simulink model "snap_fengine"  (R2016b)
settings: Solver=VariableStepDiscrete  StartTime=0.0  StopTime=10.0  RelTol=1e-3
libraries: xbsIndex_r4 x4489, casper_library_misc x36, xps_library x10, casper_library_sources x6, casper_library_delays x5, casper_library_reorder x2, casper_library_communications x1
(part 13 of 38)

== system snap_fengine/rotator/rotator3 ==
  din : Inport
  phase : Inport  Port=2
  "CORDIC 6.0 " : xbsIndex_r4/CORDIC 6.0   functional_selection=Rotate  architectural_configuration=Parallel  pipelining_mode=Optimal  data_format=SignedFraction  phase_format=Radians  input_width=18  output_width=18  round_mode=Nearest_Even  iterations=0  precision=0  compensation_scaling=No_Scale_Compensation  coarse_rotation=off  aclken=off  aresetn=off  out_tready=off  cartesian_has_tuser=off  cartesian_has_tlast=off  cartesian_tuser_width=1  phase_has_tuser=off  phase_has_tlast=off  phase_tuser_width=1  out_tlast_behv=Null  flow_control=NonBlocking  optimize_goal=Resources  trim_axipin_name=on  simulation_type=hybrid_sim  simulation_model=sysgen:cordic_v6_0  data_path_portlist={'s_axis_cartesian_tdata_imag', 's_axis_cartesian_tdata_real', 's_axis_phase_tdata_phase', 'm_axis_dout_tdata_imag', 'm_axis_dout_tdata_real', 'm_axis_dout_tdata_phase','m_axis_dout_tdata'}  ip_name=CORDIC  ip_version=6.0  dsptool_ready=true  ipcore_usecache=true  ipcore_useipmodelcache=true  wrapper_available=true  port_translation_map={ 'aclken' => 'en', 'aresetn' => 'rst' }  block_type=cordic_v6_0
      settings: infoedit=CORDIC 6.0
  Constant2 : xbsIndex_r4/Constant  const=1  gui_display_data_type=Boolean  arith_type=Boolean  n_bits=32  bin_pt=0  preci_type=Single  exp_width=8  frac_width=24  explicit_period=on  period=1  equ=P=C  opselect=C  inp2=PCIN>>17  opr=+  inp1=P  carry=CIN  dbl_ovrd=off  block_type=constant
  Constant3 : xbsIndex_r4/Constant  const=1  gui_display_data_type=Boolean  arith_type=Boolean  n_bits=32  bin_pt=0  preci_type=Single  exp_width=8  frac_width=24  explicit_period=on  period=1  equ=P=C  opselect=C  inp2=PCIN>>17  opr=+  inp1=P  carry=CIN  dbl_ovrd=off  block_type=constant
  Reinterpret : xbsIndex_r4/Reinterpret  force_arith_type=on  arith_type="Signed  (2's comp)"  force_bin_pt=on  bin_pt=16  block_type=reinterpret
  Reinterpret1 : xbsIndex_r4/Reinterpret  force_arith_type=on  arith_type="Signed  (2's comp)"  force_bin_pt=on  bin_pt=16  block_type=reinterpret
  c_to_ri : casper_library_misc/c_to_ri  n_bits=18  bin_pt=17
  ri_to_c : casper_library_misc/ri_to_c
  vld : Outport
  dout : Outport  Port=2
  wires:
  Constant2/1 -> "CORDIC 6.0 "/4
  c_to_ri/1 -> Reinterpret/1
  ri_to_c/1 -> dout/1
  phase/1 -> "CORDIC 6.0 "/5
  Constant3/1 -> "CORDIC 6.0 "/1
  "CORDIC 6.0 "/2 -> ri_to_c/2
  "CORDIC 6.0 "/1 -> vld/1
  "CORDIC 6.0 "/3 -> ri_to_c/1
  din/1 -> c_to_ri/1
  c_to_ri/2 -> Reinterpret1/1
  Reinterpret/1 -> "CORDIC 6.0 "/3
  Reinterpret1/1 -> "CORDIC 6.0 "/2

== system snap_fengine/rotator/rotator4 ==
  din : Inport
  phase : Inport  Port=2
  "CORDIC 6.0 " : xbsIndex_r4/CORDIC 6.0   functional_selection=Rotate  architectural_configuration=Parallel  pipelining_mode=Optimal  data_format=SignedFraction  phase_format=Radians  input_width=18  output_width=18  round_mode=Nearest_Even  iterations=0  precision=0  compensation_scaling=No_Scale_Compensation  coarse_rotation=off  aclken=off  aresetn=off  out_tready=off  cartesian_has_tuser=off  cartesian_has_tlast=off  cartesian_tuser_width=1  phase_has_tuser=off  phase_has_tlast=off  phase_tuser_width=1  out_tlast_behv=Null  flow_control=NonBlocking  optimize_goal=Resources  trim_axipin_name=on  simulation_type=hybrid_sim  simulation_model=sysgen:cordic_v6_0  data_path_portlist={'s_axis_cartesian_tdata_imag', 's_axis_cartesian_tdata_real', 's_axis_phase_tdata_phase', 'm_axis_dout_tdata_imag', 'm_axis_dout_tdata_real', 'm_axis_dout_tdata_phase','m_axis_dout_tdata'}  ip_name=CORDIC  ip_version=6.0  dsptool_ready=true  ipcore_usecache=true  ipcore_useipmodelcache=true  wrapper_available=true  port_translation_map={ 'aclken' => 'en', 'aresetn' => 'rst' }  block_type=cordic_v6_0
      settings: infoedit=CORDIC 6.0
  Constant2 : xbsIndex_r4/Constant  const=1  gui_display_data_type=Boolean  arith_type=Boolean  n_bits=32  bin_pt=0  preci_type=Single  exp_width=8  frac_width=24  explicit_period=on  period=1  equ=P=C  opselect=C  inp2=PCIN>>17  opr=+  inp1=P  carry=CIN  dbl_ovrd=off  block_type=constant
  Constant3 : xbsIndex_r4/Constant  const=1  gui_display_data_type=Boolean  arith_type=Boolean  n_bits=32  bin_pt=0  preci_type=Single  exp_width=8  frac_width=24  explicit_period=on  period=1  equ=P=C  opselect=C  inp2=PCIN>>17  opr=+  inp1=P  carry=CIN  dbl_ovrd=off  block_type=constant
  Reinterpret : xbsIndex_r4/Reinterpret  force_arith_type=on  arith_type="Signed  (2's comp)"  force_bin_pt=on  bin_pt=16  block_type=reinterpret
  Reinterpret1 : xbsIndex_r4/Reinterpret  force_arith_type=on  arith_type="Signed  (2's comp)"  force_bin_pt=on  bin_pt=16  block_type=reinterpret
  c_to_ri : casper_library_misc/c_to_ri  n_bits=18  bin_pt=17
  ri_to_c : casper_library_misc/ri_to_c
  vld : Outport
  dout : Outport  Port=2
  wires:
  Reinterpret1/1 -> "CORDIC 6.0 "/2
  Reinterpret/1 -> "CORDIC 6.0 "/3
  c_to_ri/2 -> Reinterpret1/1
  din/1 -> c_to_ri/1
  "CORDIC 6.0 "/3 -> ri_to_c/1
  "CORDIC 6.0 "/1 -> vld/1
  "CORDIC 6.0 "/2 -> ri_to_c/2
  Constant3/1 -> "CORDIC 6.0 "/1
  phase/1 -> "CORDIC 6.0 "/5
  ri_to_c/1 -> dout/1
  c_to_ri/1 -> Reinterpret/1
  Constant2/1 -> "CORDIC 6.0 "/4

== system snap_fengine/rotator/rotator5 ==
  din : Inport
  phase : Inport  Port=2
  "CORDIC 6.0 " : xbsIndex_r4/CORDIC 6.0   functional_selection=Rotate  architectural_configuration=Parallel  pipelining_mode=Optimal  data_format=SignedFraction  phase_format=Radians  input_width=18  output_width=18  round_mode=Nearest_Even  iterations=0  precision=0  compensation_scaling=No_Scale_Compensation  coarse_rotation=off  aclken=off  aresetn=off  out_tready=off  cartesian_has_tuser=off  cartesian_has_tlast=off  cartesian_tuser_width=1  phase_has_tuser=off  phase_has_tlast=off  phase_tuser_width=1  out_tlast_behv=Null  flow_control=NonBlocking  optimize_goal=Resources  trim_axipin_name=on  simulation_type=hybrid_sim  simulation_model=sysgen:cordic_v6_0  data_path_portlist={'s_axis_cartesian_tdata_imag', 's_axis_cartesian_tdata_real', 's_axis_phase_tdata_phase', 'm_axis_dout_tdata_imag', 'm_axis_dout_tdata_real', 'm_axis_dout_tdata_phase','m_axis_dout_tdata'}  ip_name=CORDIC  ip_version=6.0  dsptool_ready=true  ipcore_usecache=true  ipcore_useipmodelcache=true  wrapper_available=true  port_translation_map={ 'aclken' => 'en', 'aresetn' => 'rst' }  block_type=cordic_v6_0
      settings: infoedit=CORDIC 6.0
  Constant2 : xbsIndex_r4/Constant  const=1  gui_display_data_type=Boolean  arith_type=Boolean  n_bits=32  bin_pt=0  preci_type=Single  exp_width=8  frac_width=24  explicit_period=on  period=1  equ=P=C  opselect=C  inp2=PCIN>>17  opr=+  inp1=P  carry=CIN  dbl_ovrd=off  block_type=constant
  Constant3 : xbsIndex_r4/Constant  const=1  gui_display_data_type=Boolean  arith_type=Boolean  n_bits=32  bin_pt=0  preci_type=Single  exp_width=8  frac_width=24  explicit_period=on  period=1  equ=P=C  opselect=C  inp2=PCIN>>17  opr=+  inp1=P  carry=CIN  dbl_ovrd=off  block_type=constant
  Reinterpret : xbsIndex_r4/Reinterpret  force_arith_type=on  arith_type="Signed  (2's comp)"  force_bin_pt=on  bin_pt=16  block_type=reinterpret
  Reinterpret1 : xbsIndex_r4/Reinterpret  force_arith_type=on  arith_type="Signed  (2's comp)"  force_bin_pt=on  bin_pt=16  block_type=reinterpret
  c_to_ri : casper_library_misc/c_to_ri  n_bits=18  bin_pt=17
  ri_to_c : casper_library_misc/ri_to_c
  vld : Outport
  dout : Outport  Port=2
  wires:
  Constant2/1 -> "CORDIC 6.0 "/4
  c_to_ri/1 -> Reinterpret/1
  ri_to_c/1 -> dout/1
  phase/1 -> "CORDIC 6.0 "/5
  Constant3/1 -> "CORDIC 6.0 "/1
  "CORDIC 6.0 "/2 -> ri_to_c/2
  "CORDIC 6.0 "/1 -> vld/1
  "CORDIC 6.0 "/3 -> ri_to_c/1
  din/1 -> c_to_ri/1
  c_to_ri/2 -> Reinterpret1/1
  Reinterpret/1 -> "CORDIC 6.0 "/3
  Reinterpret1/1 -> "CORDIC 6.0 "/2

== system snap_fengine/rotator/rotator6 ==
  din : Inport
  phase : Inport  Port=2
  "CORDIC 6.0 " : xbsIndex_r4/CORDIC 6.0   functional_selection=Rotate  architectural_configuration=Parallel  pipelining_mode=Optimal  data_format=SignedFraction  phase_format=Radians  input_width=18  output_width=18  round_mode=Nearest_Even  iterations=0  precision=0  compensation_scaling=No_Scale_Compensation  coarse_rotation=off  aclken=off  aresetn=off  out_tready=off  cartesian_has_tuser=off  cartesian_has_tlast=off  cartesian_tuser_width=1  phase_has_tuser=off  phase_has_tlast=off  phase_tuser_width=1  out_tlast_behv=Null  flow_control=NonBlocking  optimize_goal=Resources  trim_axipin_name=on  simulation_type=hybrid_sim  simulation_model=sysgen:cordic_v6_0  data_path_portlist={'s_axis_cartesian_tdata_imag', 's_axis_cartesian_tdata_real', 's_axis_phase_tdata_phase', 'm_axis_dout_tdata_imag', 'm_axis_dout_tdata_real', 'm_axis_dout_tdata_phase','m_axis_dout_tdata'}  ip_name=CORDIC  ip_version=6.0  dsptool_ready=true  ipcore_usecache=true  ipcore_useipmodelcache=true  wrapper_available=true  port_translation_map={ 'aclken' => 'en', 'aresetn' => 'rst' }  block_type=cordic_v6_0
      settings: infoedit=CORDIC 6.0
  Constant2 : xbsIndex_r4/Constant  const=1  gui_display_data_type=Boolean  arith_type=Boolean  n_bits=32  bin_pt=0  preci_type=Single  exp_width=8  frac_width=24  explicit_period=on  period=1  equ=P=C  opselect=C  inp2=PCIN>>17  opr=+  inp1=P  carry=CIN  dbl_ovrd=off  block_type=constant
  Constant3 : xbsIndex_r4/Constant  const=1  gui_display_data_type=Boolean  arith_type=Boolean  n_bits=32  bin_pt=0  preci_type=Single  exp_width=8  frac_width=24  explicit_period=on  period=1  equ=P=C  opselect=C  inp2=PCIN>>17  opr=+  inp1=P  carry=CIN  dbl_ovrd=off  block_type=constant
  Reinterpret : xbsIndex_r4/Reinterpret  force_arith_type=on  arith_type="Signed  (2's comp)"  force_bin_pt=on  bin_pt=16  block_type=reinterpret
  Reinterpret1 : xbsIndex_r4/Reinterpret  force_arith_type=on  arith_type="Signed  (2's comp)"  force_bin_pt=on  bin_pt=16  block_type=reinterpret
  c_to_ri : casper_library_misc/c_to_ri  n_bits=18  bin_pt=17
  ri_to_c : casper_library_misc/ri_to_c
  vld : Outport
  dout : Outport  Port=2
  wires:
  Constant2/1 -> "CORDIC 6.0 "/4
  c_to_ri/1 -> Reinterpret/1
  ri_to_c/1 -> dout/1
  phase/1 -> "CORDIC 6.0 "/5
  Constant3/1 -> "CORDIC 6.0 "/1
  "CORDIC 6.0 "/2 -> ri_to_c/2
  "CORDIC 6.0 "/1 -> vld/1
  "CORDIC 6.0 "/3 -> ri_to_c/1
  din/1 -> c_to_ri/1
  c_to_ri/2 -> Reinterpret1/1
  Reinterpret/1 -> "CORDIC 6.0 "/3
  Reinterpret1/1 -> "CORDIC 6.0 "/2

== system snap_fengine/rotator/rotator7 ==
  din : Inport
  phase : Inport  Port=2
  "CORDIC 6.0 " : xbsIndex_r4/CORDIC 6.0   functional_selection=Rotate  architectural_configuration=Parallel  pipelining_mode=Optimal  data_format=SignedFraction  phase_format=Radians  input_width=18  output_width=18  round_mode=Nearest_Even  iterations=0  precision=0  compensation_scaling=No_Scale_Compensation  coarse_rotation=off  aclken=off  aresetn=off  out_tready=off  cartesian_has_tuser=off  cartesian_has_tlast=off  cartesian_tuser_width=1  phase_has_tuser=off  phase_has_tlast=off  phase_tuser_width=1  out_tlast_behv=Null  flow_control=NonBlocking  optimize_goal=Resources  trim_axipin_name=on  simulation_type=hybrid_sim  simulation_model=sysgen:cordic_v6_0  data_path_portlist={'s_axis_cartesian_tdata_imag', 's_axis_cartesian_tdata_real', 's_axis_phase_tdata_phase', 'm_axis_dout_tdata_imag', 'm_axis_dout_tdata_real', 'm_axis_dout_tdata_phase','m_axis_dout_tdata'}  ip_name=CORDIC  ip_version=6.0  dsptool_ready=true  ipcore_usecache=true  ipcore_useipmodelcache=true  wrapper_available=true  port_translation_map={ 'aclken' => 'en', 'aresetn' => 'rst' }  block_type=cordic_v6_0
      settings: infoedit=CORDIC 6.0
  Constant2 : xbsIndex_r4/Constant  const=1  gui_display_data_type=Boolean  arith_type=Boolean  n_bits=32  bin_pt=0  preci_type=Single  exp_width=8  frac_width=24  explicit_period=on  period=1  equ=P=C  opselect=C  inp2=PCIN>>17  opr=+  inp1=P  carry=CIN  dbl_ovrd=off  block_type=constant
  Constant3 : xbsIndex_r4/Constant  const=1  gui_display_data_type=Boolean  arith_type=Boolean  n_bits=32  bin_pt=0  preci_type=Single  exp_width=8  frac_width=24  explicit_period=on  period=1  equ=P=C  opselect=C  inp2=PCIN>>17  opr=+  inp1=P  carry=CIN  dbl_ovrd=off  block_type=constant
  Reinterpret : xbsIndex_r4/Reinterpret  force_arith_type=on  arith_type="Signed  (2's comp)"  force_bin_pt=on  bin_pt=16  block_type=reinterpret
  Reinterpret1 : xbsIndex_r4/Reinterpret  force_arith_type=on  arith_type="Signed  (2's comp)"  force_bin_pt=on  bin_pt=16  block_type=reinterpret
  c_to_ri : casper_library_misc/c_to_ri  n_bits=18  bin_pt=17
  ri_to_c : casper_library_misc/ri_to_c
  vld : Outport
  dout : Outport  Port=2
  wires:
  Reinterpret1/1 -> "CORDIC 6.0 "/2
  Reinterpret/1 -> "CORDIC 6.0 "/3
  c_to_ri/2 -> Reinterpret1/1
  din/1 -> c_to_ri/1
  "CORDIC 6.0 "/3 -> ri_to_c/1
  "CORDIC 6.0 "/1 -> vld/1
  "CORDIC 6.0 "/2 -> ri_to_c/2
  Constant3/1 -> "CORDIC 6.0 "/1
  phase/1 -> "CORDIC 6.0 "/5
  ri_to_c/1 -> dout/1
  c_to_ri/1 -> Reinterpret/1
  Constant2/1 -> "CORDIC 6.0 "/4

== system snap_fengine/sync/arm ==
  sim_1 : Inport
  io_delay : xbsIndex_r4/Delay  rst=off  infoeditControl=Selection of Reset will increase slice count due to use of real FFs and instead of SRLs  en=off  latency=0  reg_retiming=on  dbl_ovrd=off  block_type=delay
  reint1 : xbsIndex_r4/Reinterpret  force_arith_type=on  arith_type=Unsigned  force_bin_pt=on  bin_pt=0  block_type=reinterpret
  slice_reg : xbsIndex_r4/Slice  nbits=32  boolean_output=off  mode=Lower Bit Location + Width  bit1=0  base1=MSB of Input  bit0=0  base0=LSB of Input  dbl_ovrd=off  block_type=slice
  snap_fengine_sync_arm_user_data_out : xbsIndex_r4/Gateway In  gui_display_data_type=Fixed-point  arith_type=Unsigned  n_bits=32  bin_pt=0  preci_type=Single  exp_width=8  frac_width=24  rows=1  columns=1  quantization="Round  (unbiased: +/- Inf)"  overflow=Saturate  period=1  UseAsADC=off  ADCChannel='1'  interface=None  automatic_assignment=on  address_offset=hex2dec('00')  intf_name=''  intf_description=''  default_value=0  timing_constraint=None  locs_specified=off  LOCs={}  io_standard={}  inherit_from_input=off  hdl_port=on  dbl_ovrd=off  block_type=gatewayin
  in_reg : Outport
  wires:
  snap_fengine_sync_arm_user_data_out/1 -> io_delay/1
  sim_1/1 -> snap_fengine_sync_arm_user_data_out/1
  io_delay/1 -> slice_reg/1
  slice_reg/1 -> reint1/1
  reint1/1 -> in_reg/1

== system snap_fengine/sync/count ==
  out_reg : Inport
  assert_reg : xbsIndex_r4/Assert  assert_type=on  type_source=Explicitly  gui_display_data_type=Fixed-point  arith_type=Unsigned  n_bits=32  bin_pt=0  preci_type=Single  exp_width=8  frac_width=24  assert_rate=off  rate_source=Explicitly  period=1  output_port=on  block_type=assert
  cast_gw : xbsIndex_r4/Convert  gui_display_data_type=Fixed-point  arith_type=Unsigned  n_bits=32  bin_pt=0  float_type=Single  exp_bits=8  fraction_bits=24  quantization=Truncate  overflow=Wrap  en=off  latency=1  pipeline=off  dbl_ovrd=off  block_type=convert
  io_delay : xbsIndex_r4/Delay  rst=off  infoeditControl=Selection of Reset will increase slice count due to use of real FFs and instead of SRLs  en=off  latency=0  reg_retiming=on  dbl_ovrd=off  block_type=delay
  reint1 : xbsIndex_r4/Reinterpret  force_arith_type=on  arith_type=Unsigned  force_bin_pt=on  bin_pt=0  block_type=reinterpret
  snap_fengine_sync_count_user_data_in : xbsIndex_r4/Gateway Out  inherit_from_input=off  hdl_port=on  rows=1  columns=1  UseAsDAC=off  DACChannel='1'  interface=None  automatic_assignment=on  address_offset=hex2dec('00')  intf_name=''  intf_description=''  timing_constraint=None  locs_specified=off  LOCs={}  io_standard={}  block_type=gatewayout
  sim_out : Outport
  wires:
  io_delay/1 -> cast_gw/1
  cast_gw/1 -> snap_fengine_sync_count_user_data_in/1
  snap_fengine_sync_count_user_data_in/1 -> sim_out/1
  out_reg/1 -> assert_reg/1
  assert_reg/1 -> reint1/1
  reint1/1 -> io_delay/1

== system snap_fengine/sync/ed ==
  in : Inport
  Delay : xbsIndex_r4/Delay  rst=off  infoeditControl=Selection of Reset will increase slice count due to use of real FFs and instead of SRLs  en=off  latency=1  reg_retiming=off  dbl_ovrd=off  block_type=delay
      settings: xl_area=[0, 0, 0, 0, 0, 0, 0]
  Inverter : xbsIndex_r4/Inverter  en=off  latency=0  dbl_ovrd=off  block_type=inv
      settings: xl_area=[0, 0, 0, 0, 0, 0, 0]
  edge_op : xbsIndex_r4/Logical  logical_function=NOR  inputs=2  en=off  latency=0  precision=Full  arith_type=Unsigned  n_bits=8  bin_pt=2  align_bp=on  dbl_ovrd=off  block_type=logical
      settings: xl_area=[0, 0, 0, 0, 0, 0, 0]
  out : Outport
  wires:
  Inverter/1 -> edge_op/1
  edge_op/1 -> out/1
  in/1 -> Inverter/1, Delay/1
  Delay/1 -> edge_op/2

== system snap_fengine/sync/ed1 ==
  in : Inport
  Delay : xbsIndex_r4/Delay  rst=off  infoeditControl=Selection of Reset will increase slice count due to use of real FFs and instead of SRLs  en=off  latency=1  reg_retiming=off  dbl_ovrd=off  block_type=delay
      settings: xl_area=[0, 0, 0, 0, 0, 0, 0]
  Inverter : xbsIndex_r4/Inverter  en=off  latency=0  dbl_ovrd=off  block_type=inv
      settings: xl_area=[0, 0, 0, 0, 0, 0, 0]
  edge_op : xbsIndex_r4/Logical  logical_function=AND  inputs=2  en=off  latency=0  precision=Full  arith_type=Unsigned  n_bits=8  bin_pt=2  align_bp=on  dbl_ovrd=off  block_type=logical
      settings: xl_area=[0, 0, 0, 0, 0, 0, 0]
  out : Outport
  wires:
  Inverter/1 -> edge_op/1
  edge_op/1 -> out/1
  in/1 -> Inverter/1, Delay/1
  Delay/1 -> edge_op/2

== system snap_fengine/sync/ed2 ==
  in : Inport
  Delay : xbsIndex_r4/Delay  rst=off  infoeditControl=Selection of Reset will increase slice count due to use of real FFs and instead of SRLs  en=off  latency=1  reg_retiming=off  dbl_ovrd=off  block_type=delay
      settings: xl_area=[0, 0, 0, 0, 0, 0, 0]
  Inverter : xbsIndex_r4/Inverter  en=off  latency=0  dbl_ovrd=off  block_type=inv
      settings: xl_area=[0, 0, 0, 0, 0, 0, 0]
  edge_op : xbsIndex_r4/Logical  logical_function=NOR  inputs=2  en=off  latency=0  precision=Full  arith_type=Unsigned  n_bits=8  bin_pt=2  align_bp=on  dbl_ovrd=off  block_type=logical
      settings: xl_area=[0, 0, 0, 0, 0, 0, 0]
  out : Outport
  wires:
  Inverter/1 -> edge_op/1
  edge_op/1 -> out/1
  in/1 -> Inverter/1, Delay/1
  Delay/1 -> edge_op/2

== system snap_fengine/sync/ed3 ==
  in : Inport
  Delay : xbsIndex_r4/Delay  rst=off  infoeditControl=Selection of Reset will increase slice count due to use of real FFs and instead of SRLs  en=off  latency=1  reg_retiming=off  dbl_ovrd=off  block_type=delay
      settings: xl_area=[0, 0, 0, 0, 0, 0, 0]
  Inverter : xbsIndex_r4/Inverter  en=off  latency=0  dbl_ovrd=off  block_type=inv
      settings: xl_area=[0, 0, 0, 0, 0, 0, 0]
  edge_op : xbsIndex_r4/Logical  logical_function=NOR  inputs=2  en=off  latency=0  precision=Full  arith_type=Unsigned  n_bits=8  bin_pt=2  align_bp=on  dbl_ovrd=off  block_type=logical
      settings: xl_area=[0, 0, 0, 0, 0, 0, 0]
  out : Outport
  wires:
  Inverter/1 -> edge_op/1
  edge_op/1 -> out/1
  in/1 -> Inverter/1, Delay/1
  Delay/1 -> edge_op/2

== system snap_fengine/sync/ed4 ==
  in : Inport
  Delay : xbsIndex_r4/Delay  rst=off  infoeditControl=Selection of Reset will increase slice count due to use of real FFs and instead of SRLs  en=off  latency=1  reg_retiming=off  dbl_ovrd=off  block_type=delay
      settings: xl_area=[0, 0, 0, 0, 0, 0, 0]
  Inverter : xbsIndex_r4/Inverter  en=off  latency=0  dbl_ovrd=off  block_type=inv
      settings: xl_area=[0, 0, 0, 0, 0, 0, 0]
  edge_op : xbsIndex_r4/Logical  logical_function=NOR  inputs=2  en=off  latency=0  precision=Full  arith_type=Unsigned  n_bits=8  bin_pt=2  align_bp=on  dbl_ovrd=off  block_type=logical
      settings: xl_area=[0, 0, 0, 0, 0, 0, 0]
  out : Outport
  wires:
  Inverter/1 -> edge_op/1
  edge_op/1 -> out/1
  in/1 -> Inverter/1, Delay/1
  Delay/1 -> edge_op/2

== system snap_fengine/sync/ed5 ==
  in : Inport
  Delay : xbsIndex_r4/Delay  rst=off  infoeditControl=Selection of Reset will increase slice count due to use of real FFs and instead of SRLs  en=off  latency=1  reg_retiming=off  dbl_ovrd=off  block_type=delay
      settings: xl_area=[0, 0, 0, 0, 0, 0, 0]
  Inverter : xbsIndex_r4/Inverter  en=off  latency=0  dbl_ovrd=off  block_type=inv
      settings: xl_area=[0, 0, 0, 0, 0, 0, 0]
  edge_op : xbsIndex_r4/Logical  logical_function=NOR  inputs=2  en=off  latency=0  precision=Full  arith_type=Unsigned  n_bits=8  bin_pt=2  align_bp=on  dbl_ovrd=off  block_type=logical
      settings: xl_area=[0, 0, 0, 0, 0, 0, 0]
  out : Outport
  wires:
  Inverter/1 -> edge_op/1
  edge_op/1 -> out/1
  in/1 -> Inverter/1, Delay/1
  Delay/1 -> edge_op/2

== system snap_fengine/sync/period ==
  out_reg : Inport
  assert_reg : xbsIndex_r4/Assert  assert_type=on  type_source=Explicitly  gui_display_data_type=Fixed-point  arith_type=Unsigned  n_bits=32  bin_pt=0  preci_type=Single  exp_width=8  frac_width=24  assert_rate=off  rate_source=Explicitly  period=1  output_port=on  block_type=assert
  cast_gw : xbsIndex_r4/Convert  gui_display_data_type=Fixed-point  arith_type=Unsigned  n_bits=32  bin_pt=0  float_type=Single  exp_bits=8  fraction_bits=24  quantization=Truncate  overflow=Wrap  en=off  latency=1  pipeline=off  dbl_ovrd=off  block_type=convert
  io_delay : xbsIndex_r4/Delay  rst=off  infoeditControl=Selection of Reset will increase slice count due to use of real FFs and instead of SRLs  en=off  latency=0  reg_retiming=on  dbl_ovrd=off  block_type=delay
  reint1 : xbsIndex_r4/Reinterpret  force_arith_type=on  arith_type=Unsigned  force_bin_pt=on  bin_pt=0  block_type=reinterpret
  snap_fengine_sync_period_user_data_in : xbsIndex_r4/Gateway Out  inherit_from_input=off  hdl_port=on  rows=1  columns=1  UseAsDAC=off  DACChannel='1'  interface=None  automatic_assignment=on  address_offset=hex2dec('00')  intf_name=''  intf_description=''  timing_constraint=None  locs_specified=off  LOCs={}  io_standard={}  block_type=gatewayout
  sim_out : Outport
  wires:
  io_delay/1 -> cast_gw/1
  cast_gw/1 -> snap_fengine_sync_period_user_data_in/1
  snap_fengine_sync_period_user_data_in/1 -> sim_out/1
  out_reg/1 -> assert_reg/1
  assert_reg/1 -> reint1/1
  reint1/1 -> io_delay/1

== system snap_fengine/sync/uptime ==
  out_reg : Inport
  assert_reg : xbsIndex_r4/Assert  assert_type=on  type_source=Explicitly  gui_display_data_type=Fixed-point  arith_type=Unsigned  n_bits=32  bin_pt=0  preci_type=Single  exp_width=8  frac_width=24  assert_rate=off  rate_source=Explicitly  period=1  output_port=on  block_type=assert
  cast_gw : xbsIndex_r4/Convert  gui_display_data_type=Fixed-point  arith_type=Unsigned  n_bits=32  bin_pt=0  float_type=Single  exp_bits=8  fraction_bits=24  quantization=Truncate  overflow=Wrap  en=off  latency=1  pipeline=off  dbl_ovrd=off  block_type=convert
  io_delay : xbsIndex_r4/Delay  rst=off  infoeditControl=Selection of Reset will increase slice count due to use of real FFs and instead of SRLs  en=off  latency=0  reg_retiming=on  dbl_ovrd=off  block_type=delay
  reint1 : xbsIndex_r4/Reinterpret  force_arith_type=on  arith_type=Unsigned  force_bin_pt=on  bin_pt=0  block_type=reinterpret
  snap_fengine_sync_uptime_user_data_in : xbsIndex_r4/Gateway Out  inherit_from_input=off  hdl_port=on  rows=1  columns=1  UseAsDAC=off  DACChannel='1'  interface=None  automatic_assignment=on  address_offset=hex2dec('00')  intf_name=''  intf_description=''  timing_constraint=None  locs_specified=off  LOCs={}  io_standard={}  block_type=gatewayout
  sim_out : Outport
  wires:
  io_delay/1 -> cast_gw/1
  cast_gw/1 -> snap_fengine_sync_uptime_user_data_in/1
  snap_fengine_sync_uptime_user_data_in/1 -> sim_out/1
  out_reg/1 -> assert_reg/1
  assert_reg/1 -> reint1/1
  reint1/1 -> io_delay/1

== system snap_fengine/timebase/sync_period ==
  sim_1 : Inport
  io_delay : xbsIndex_r4/Delay  rst=off  infoeditControl=Selection of Reset will increase slice count due to use of real FFs and instead of SRLs  en=off  latency=0  reg_retiming=on  dbl_ovrd=off  block_type=delay
  reint1 : xbsIndex_r4/Reinterpret  force_arith_type=on  arith_type=Unsigned  force_bin_pt=on  bin_pt=0  block_type=reinterpret
  slice_reg : xbsIndex_r4/Slice  nbits=32  boolean_output=off  mode=Lower Bit Location + Width  bit1=0  base1=MSB of Input  bit0=0  base0=LSB of Input  dbl_ovrd=off  block_type=slice
  snap_fengine_timebase_sync_period_user_data_out : xbsIndex_r4/Gateway In  gui_display_data_type=Fixed-point  arith_type=Unsigned  n_bits=32  bin_pt=0  preci_type=Single  exp_width=8  frac_width=24  rows=1  columns=1  quantization="Round  (unbiased: +/- Inf)"  overflow=Saturate  period=1  UseAsADC=off  ADCChannel='1'  interface=None  automatic_assignment=on  address_offset=hex2dec('00')  intf_name=''  intf_description=''  default_value=0  timing_constraint=None  locs_specified=off  LOCs={}  io_standard={}  inherit_from_input=off  hdl_port=on  dbl_ovrd=off  block_type=gatewayin
  in_reg : Outport
  wires:
  snap_fengine_timebase_sync_period_user_data_out/1 -> io_delay/1
  sim_1/1 -> snap_fengine_timebase_sync_period_user_data_out/1
  io_delay/1 -> slice_reg/1
  slice_reg/1 -> reint1/1
  reint1/1 -> in_reg/1

== system snap_fengine/timebase/timing ==
  note: On arm rising edge
      | raises armed till specified
      | number of ppss seen.
  note: Generates sync one
      | clk cycle after rst
      | lowered. Syncs
      | produced with
      | specified period
  arm : Inport
  data_in : Inport  Port=2
  sync_period : Inport  Port=3
  pps_in : Inport  Port=4
  Delay : xbsIndex_r4/Delay  rst=off  infoeditControl=Selection of Reset will increase slice count due to use of real FFs and instead of SRLs  en=off  latency=1  reg_retiming=off  dbl_ovrd=off  block_type=delay
      settings: block_version=11.4
  Delay1 : xbsIndex_r4/Delay  rst=off  infoeditControl=Selection of Reset will increase slice count due to use of real FFs and instead of SRLs  en=off  latency=1  reg_retiming=off  dbl_ovrd=off  block_type=delay
      settings: block_version=11.4
  Delay2 : xbsIndex_r4/Delay  rst=off  infoeditControl=Selection of Reset will increase slice count due to use of real FFs and instead of SRLs  en=off  latency=1  reg_retiming=off  dbl_ovrd=off  block_type=delay
      settings: block_version=11.4
  Slice : xbsIndex_r4/Slice  nbits=sync_gen_bits  boolean_output=off  mode=Lower Bit Location + Width  bit1=0  base1=MSB of Input  bit0=0  base0=LSB of Input  dbl_ovrd=off  block_type=slice
      settings: infoedit="Extracts a given range of bits from each input sample and presents it at the output.  The output type is ordinarily unsigned with binary point at zero, but can be Boolean when the slice is one bit wide.<P><P>Hardware notes: In hardware this block costs nothing."  block_version=10.1.3
  rst_gen : Subsystem  mask{reset_period=reset_period}
      mask prompts: reset_period "Min period of reset (pps pulses)"
      mask init:
      | %reset_period = eval(get_param(gcb,'reset_period'))
      | %bits = ceil(log2(reset_period))
      | %set_param([gcb,'/Counter'],'n_bits',num2str(bits));
      | %set_param([gcb,'/Counter'],'start_count', num2str(reset_period))
      | %set_param([gcb,'/Constant'],'n_bits',num2str(bits));
  sync_gen : Subsystem  mask{sync_gen_bits=sync_gen_bits}
      mask prompts: sync_gen_bits "Size of sync generator counter"
  armed : Outport
  sync : Outport  Port=2
  data_out : Outport  Port=3
  wires:
  arm/1 -> rst_gen/1(arm)
  data_in/1 -> rst_gen/3(din)
  pps_in/1 -> rst_gen/2(pps_in)
  sync_period/1 -> Slice/1
  rst_gen/1(mrst) -> Delay2/1, sync_gen/1(rst)
  sync_gen/1(sync) -> Delay1/1
  Slice/1 -> sync_gen/2(sync_period)
  sync_gen/2(dout) -> Delay/1
  rst_gen/2(dout) -> sync_gen/3(din)
  Delay/1 -> data_out/1
  Delay1/1 -> sync/1
  Delay2/1 -> armed/1

== system snap_fengine/chan_reorder/reorder1/addr_expand ==
  bus_in : Inport
  reinterpret1 : xbsIndex_r4/Reinterpret  force_arith_type=on  arith_type=Unsigned  force_bin_pt=on  bin_pt=0  block_type=reinterpret
  slice1 : xbsIndex_r4/Slice  nbits=2  boolean_output=off  mode=Upper Bit Location + Width  bit1=0  base1=MSB of Input  bit0=0  base0=LSB of Input  dbl_ovrd=off  block_type=slice
  msb_lsb_out1 : Outport
  wires:
  bus_in/1 -> slice1/1
  slice1/1 -> reinterpret1/1
  reinterpret1/1 -> msb_lsb_out1/1

== system snap_fengine/chan_reorder/reorder1/addr_replicate ==
  in : Inport
  bussify : Subsystem  AncestorBlock=casper_library_flow_control/bus_create  mask(bus_create){inputNum=1}
      mask prompts: inputNum "Number of inputs:"
      mask init:
      | bus_create_init(gcb,...
      |     'inputNum', inputNum);
  out : Outport
  wires:
  bussify/1(bus_out) -> out/1
  in/1 -> bussify/1(in1)

== system snap_fengine/chan_reorder/reorder1/we_expand ==
  bus_in : Inport
  slice1 : xbsIndex_r4/Slice  nbits=1  boolean_output=on  mode=Upper Bit Location + Width  bit1=0  base1=MSB of Input  bit0=0  base0=LSB of Input  dbl_ovrd=off  block_type=slice
  msb_lsb_out1 : Outport
  wires:
  slice1/1 -> msb_lsb_out1/1
  bus_in/1 -> slice1/1

== system snap_fengine/chan_reorder/reorder1/we_replicate ==
  in : Inport
  bussify : Subsystem  AncestorBlock=casper_library_flow_control/bus_create  mask(bus_create){inputNum=1}
      mask prompts: inputNum "Number of inputs:"
      mask init:
      | bus_create_init(gcb,...
      |     'inputNum', inputNum);
  out : Outport
  wires:
  bussify/1(bus_out) -> out/1
  in/1 -> bussify/1(in1)

== system snap_fengine/chan_reorder/reorder2/addr_expand ==
  bus_in : Inport
  reinterpret1 : xbsIndex_r4/Reinterpret  force_arith_type=on  arith_type=Unsigned  force_bin_pt=on  bin_pt=0  block_type=reinterpret
  slice1 : xbsIndex_r4/Slice  nbits=14  boolean_output=off  mode=Upper Bit Location + Width  bit1=0  base1=MSB of Input  bit0=0  base0=LSB of Input  dbl_ovrd=off  block_type=slice
  msb_lsb_out1 : Outport
  wires:
  bus_in/1 -> slice1/1
  slice1/1 -> reinterpret1/1
  reinterpret1/1 -> msb_lsb_out1/1

== system snap_fengine/chan_reorder/reorder2/addr_replicate ==
  in : Inport
  bussify : Subsystem  AncestorBlock=casper_library_flow_control/bus_create  mask(bus_create){inputNum=1}
      mask prompts: inputNum "Number of inputs:"
      mask init:
      | bus_create_init(gcb,...
      |     'inputNum', inputNum);
  out : Outport
  wires:
  in/1 -> bussify/1(in1)
  bussify/1(bus_out) -> out/1

== system snap_fengine/chan_reorder/reorder2/buf0 ==
  addr : Inport
  din : Inport  Port=2
  we : Inport  Port=3
  bram{0..63} (64 alike) : xbsIndex_r4/Single Port RAM  depth=16384  initVector=getfield(get_param(gcb, 'UserData'), 'initVector')  distributed_mem=Block RAM  write_mode=Read Before Write  rst=off  init_reg=0  en=off  latency=3  optimize=Speed  dbl_ovrd=off  block_type=spram
  ddin : xbsIndex_r4/Delay  rst=off  infoeditControl=Selection of Reset will increase slice count due to use of real FFs and instead of SRLs  en=off  latency=2  reg_retiming=on  dbl_ovrd=off  block_type=delay
  debus_addr : Subsystem  AncestorBlock=casper_library_flow_control/bus_expand  mask(bus_expand){mode=divisions of equal size, outputNum=64, outputWidth=[14 14 14 14 14 14 14 14 14 14 14 14 14 14 14 14 14 14 14 14 14 14 14 14 14 14 14 14 14 14 14 14 14 14 14 14 14 14 14 14 14 14 14 14 14 14 14 14 14 14 14 14 14 14 14 14 14 14 14 14 14 14 14 14], outputBinaryPt=[0 0 0 0 0 0 0 0 0 0 0 0 0 0 0 0 0 0 0 0 0 0 0 0 0 0 0 0 0 0 0 0 0 0 0 0 0 0 0 0 0 0 0 0 0 0 0 0 0 0 0 0 0 0 0 0 0 0 0 0 0 0 0 0], outputArithmeticType=[0 0 0 0 0 0 0 0 0 0 0 0 0 0 0 0 0 0 0 0 0 0 0 0 0 0 0 0 0 0 0 0 0 0 0 0 0 0 0 0 0 0 0 0 0 0 0 0 0 0 0 0 0 0 0 0 0 0 0 0 0 0 0 0], show_format=on, outputToWorkspace=off, variablePrefix=, outputToModelAsWell=on}
      mask prompts: outputNum "Number of outputs:"; outputWidth "Output width:"; outputBinaryPt "Output binary point position:"; outputArithmeticType "Output arithmetic type (ufix=0, fix=1, bool=2):"; show_format "Print format string?"; outputToWorkspace "Output to workspace?"; variablePrefix "Variable name prefix:"; outputToModelAsWell "Output to model as well?"
      mask help:
      | Expands a 'bus' made using a bus_create or Xilinx
      | concat block.
      | The input will be divided into the specified number
      | of outputs with the specified arithmetic types.
      | Divisions are made from most significant bit.
      mask init: same as snap_fengine/chan_reorder/bus_expand
      settings: AttributesFormatString=64 outputs: uf14.0,uf14.0,uf14.0,uf14.0,uf14.0,uf14.0,uf14.0,uf14.0,uf14.0,uf14.0,uf14.0,uf14.0,uf14.0,uf14.0,uf14.0,uf14.0,uf14.0,uf14.0,uf14.0,uf14.0,uf14.0,uf14.0,uf14.0,uf14.0,uf14.0,uf14.0,uf14.0,uf14.0,uf14.0,uf14.0,uf14.0,uf14.0,uf14.0,uf14.0,uf14.0,uf14.0,uf14.0,uf14.0,uf14.0,uf14.0,uf14.0,uf14.0,uf14.0,uf14.0,uf14.0,uf14.0,uf14.0,uf14.0,uf14.0,uf14.0,uf14.0,uf14.0,uf14.0,uf14.0,uf14.0,uf14.0,uf14.0,uf14.0,uf14.0,uf14.0,uf14.0,uf14.0,uf14.0,uf14.0,
      mask TypeOptions mode: divisions of equal size | divisions of arbitrary size
      mask Callback mode: bus_expand_callback();
      mask Callback outputWidth: bus_expand_callback();
      mask Callback outputToWorkspace: bus_expand_callback();
  debus_din : Subsystem  AncestorBlock=casper_library_flow_control/bus_expand  mask(bus_expand){mode=divisions of arbitrary size, outputNum=1, outputWidth=[1 1 1 1 1 1 1 1 1 1 1 1 1 1 1 1 1 1 1 1 1 1 1 1 1 1 1 1 1 1 1 1 1 1 1 1 1 1 1 1 1 1 1 1 1 1 1 1 1 1 1 1 1 1 1 1 1 1 1 1 1 1 1 1], outputBinaryPt=[0 0 0 0 0 0 0 0 0 0 0 0 0 0 0 0 0 0 0 0 0 0 0 0 0 0 0 0 0 0 0 0 0 0 0 0 0 0 0 0 0 0 0 0 0 0 0 0 0 0 0 0 0 0 0 0 0 0 0 0 0 0 0 0], outputArithmeticType=[0 0 0 0 0 0 0 0 0 0 0 0 0 0 0 0 0 0 0 0 0 0 0 0 0 0 0 0 0 0 0 0 0 0 0 0 0 0 0 0 0 0 0 0 0 0 0 0 0 0 0 0 0 0 0 0 0 0 0 0 0 0 0 0], show_format=on, outputToWorkspace=off, variablePrefix=, outputToModelAsWell=on}
      mask prompts: outputNum "Number of outputs:"; outputWidth "Output width [msb ... lsb]:"; outputBinaryPt "Output binary point position [msb ... lsb]:"; outputArithmeticType "Output arithmetic type (ufix=0, fix=1, bool=2) [msb ... lsb]:"; show_format "Print format string?"; outputToWorkspace "Output to workspace?"; variablePrefix "Variable name prefix:"; outputToModelAsWell "Output to model as well?"
      mask help:
      | Expands a 'bus' made using a bus_create or Xilinx
      | concat block.
      | The input will be divided into the specified number
      | of outputs with the specified arithmetic types.
      | Divisions are made from most significant bit.
      mask init: same as snap_fengine/chan_reorder/bus_expand
      settings: AttributesFormatString=64 outputs: uf1.0,uf1.0,uf1.0,uf1.0,uf1.0,uf1.0,uf1.0,uf1.0,uf1.0,uf1.0,uf1.0,uf1.0,uf1.0,uf1.0,uf1.0,uf1.0,uf1.0,uf1.0,uf1.0,uf1.0,uf1.0,uf1.0,uf1.0,uf1.0,uf1.0,uf1.0,uf1.0,uf1.0,uf1.0,uf1.0,uf1.0,uf1.0,uf1.0,uf1.0,uf1.0,uf1.0,uf1.0,uf1.0,uf1.0,uf1.0,uf1.0,uf1.0,uf1.0,uf1.0,uf1.0,uf1.0,uf1.0,uf1.0,uf1.0,uf1.0,uf1.0,uf1.0,uf1.0,uf1.0,uf1.0,uf1.0,uf1.0,uf1.0,uf1.0,uf1.0,uf1.0,uf1.0,uf1.0,uf1.0,
      mask TypeOptions mode: divisions of equal size | divisions of arbitrary size
      mask Callback mode: bus_expand_callback();
      mask Callback outputWidth: bus_expand_callback();
      mask Callback outputToWorkspace: bus_expand_callback();
  debus_we : Subsystem  AncestorBlock=casper_library_flow_control/bus_expand  mask(bus_expand){mode=divisions of equal size, outputNum=64, outputWidth=[1 1 1 1 1 1 1 1 1 1 1 1 1 1 1 1 1 1 1 1 1 1 1 1 1 1 1 1 1 1 1 1 1 1 1 1 1 1 1 1 1 1 1 1 1 1 1 1 1 1 1 1 1 1 1 1 1 1 1 1 1 1 1 1], outputBinaryPt=[0 0 0 0 0 0 0 0 0 0 0 0 0 0 0 0 0 0 0 0 0 0 0 0 0 0 0 0 0 0 0 0 0 0 0 0 0 0 0 0 0 0 0 0 0 0 0 0 0 0 0 0 0 0 0 0 0 0 0 0 0 0 0 0], outputArithmeticType=[2 2 2 2 2 2 2 2 2 2 2 2 2 2 2 2 2 2 2 2 2 2 2 2 2 2 2 2 2 2 2 2 2 2 2 2 2 2 2 2 2 2 2 2 2 2 2 2 2 2 2 2 2 2 2 2 2 2 2 2 2 2 2 2], show_format=on, outputToWorkspace=off, variablePrefix=, outputToModelAsWell=on}
      mask prompts: outputNum "Number of outputs:"; outputWidth "Output width:"; outputBinaryPt "Output binary point position:"; outputArithmeticType "Output arithmetic type (ufix=0, fix=1, bool=2):"; show_format "Print format string?"; outputToWorkspace "Output to workspace?"; variablePrefix "Variable name prefix:"; outputToModelAsWell "Output to model as well?"
      mask help:
      | Expands a 'bus' made using a bus_create or Xilinx
      | concat block.
      | The input will be divided into the specified number
      | of outputs with the specified arithmetic types.
      | Divisions are made from most significant bit.
      mask init: same as snap_fengine/chan_reorder/bus_expand
      settings: AttributesFormatString=64 outputs: b,b,b,b,b,b,b,b,b,b,b,b,b,b,b,b,b,b,b,b,b,b,b,b,b,b,b,b,b,b,b,b,b,b,b,b,b,b,b,b,b,b,b,b,b,b,b,b,b,b,b,b,b,b,b,b,b,b,b,b,b,b,b,b,
      mask TypeOptions mode: divisions of equal size | divisions of arbitrary size
      mask Callback mode: bus_expand_callback();
      mask Callback outputWidth: bus_expand_callback();
      mask Callback outputToWorkspace: bus_expand_callback();
  din_bussify : Subsystem  AncestorBlock=casper_library_flow_control/bus_create  mask(bus_create){inputNum=64}
      mask prompts: inputNum "Number of inputs:"
      mask init:
      | bus_create_init(gcb,...
      |     'inputNum', inputNum);
  rep_addr : Subsystem  AncestorBlock=casper_library_bus/bus_replicate  mask(bus_replicate){replication=64, latency=2, misc=off, implementation=core}
      mask prompts: replication "replication factor"; misc "misc support"; implementation "delay implementation"
      mask help: Output bus formed by replicating input bus a number of times
      mask init:
      | bus_replicate_init(gcb, ...
      |     'replication', replication, ...
      |     'latency', latency, ...
      |     'implementation', implementation, ...
      |     'misc', misc);
      mask TypeOptions implementation: core | behavioral
  rep_we : Subsystem  AncestorBlock=casper_library_bus/bus_replicate  mask(bus_replicate){replication=64, latency=2, misc=off, implementation=core}
      mask prompts: replication "replication factor"; misc "misc support"; implementation "delay implementation"
      mask help: Output bus formed by replicating input bus a number of times
      mask init:
      | bus_replicate_init(gcb, ...
      |     'replication', replication, ...
      |     'latency', latency, ...
      |     'implementation', implementation, ...
      |     'misc', misc);
      mask TypeOptions implementation: core | behavioral
  dout : Outport
  wires:
  addr/1 -> rep_addr/1(in)
  din/1 -> ddin/1
  we/1 -> rep_we/1(in)
  rep_addr/1(out) -> debus_addr/1(bus_in)
  ddin/1 -> debus_din/1(bus_in)
  rep_we/1(out) -> debus_we/1(bus_in)
  debus_addr/1(msb_out64) -> bram0/1
  debus_din/1(msb_out64) -> bram0/2
  debus_we/1(msb_out64) -> bram0/3
  debus_addr/2(out63) -> bram1/1
  debus_din/2(out63) -> bram1/2
  debus_we/2(out63) -> bram1/3
  debus_addr/3(out62) -> bram2/1
  debus_din/3(out62) -> bram2/2
  debus_we/3(out62) -> bram2/3
  debus_addr/4(out61) -> bram3/1
  debus_din/4(out61) -> bram3/2
  debus_we/4(out61) -> bram3/3
  debus_addr/5(out60) -> bram4/1
  debus_din/5(out60) -> bram4/2
  debus_we/5(out60) -> bram4/3
  debus_addr/6(out59) -> bram5/1
  debus_din/6(out59) -> bram5/2
  debus_we/6(out59) -> bram5/3
  debus_addr/7(out58) -> bram6/1
  debus_din/7(out58) -> bram6/2
  debus_we/7(out58) -> bram6/3
  debus_addr/8(out57) -> bram7/1
  debus_din/8(out57) -> bram7/2
  debus_we/8(out57) -> bram7/3
  debus_addr/9(out56) -> bram8/1
  debus_din/9(out56) -> bram8/2
  debus_we/9(out56) -> bram8/3
  debus_addr/10(out55) -> bram9/1
  debus_din/10(out55) -> bram9/2
  debus_we/10(out55) -> bram9/3
  debus_addr/11(out54) -> bram10/1
  debus_din/11(out54) -> bram10/2
  debus_we/11(out54) -> bram10/3
  debus_addr/12(out53) -> bram11/1
  debus_din/12(out53) -> bram11/2
  debus_we/12(out53) -> bram11/3
  debus_addr/13(out52) -> bram12/1
  debus_din/13(out52) -> bram12/2
  debus_we/13(out52) -> bram12/3
  debus_addr/14(out51) -> bram13/1
  debus_din/14(out51) -> bram13/2
  debus_we/14(out51) -> bram13/3
  debus_addr/15(out50) -> bram14/1
  debus_din/15(out50) -> bram14/2
  debus_we/15(out50) -> bram14/3
  debus_addr/16(out49) -> bram15/1
  debus_din/16(out49) -> bram15/2
  debus_we/16(out49) -> bram15/3
  debus_addr/17(out48) -> bram16/1
  debus_din/17(out48) -> bram16/2
  debus_we/17(out48) -> bram16/3
  debus_addr/18(out47) -> bram17/1
  debus_din/18(out47) -> bram17/2
  debus_we/18(out47) -> bram17/3
  debus_addr/19(out46) -> bram18/1
  debus_din/19(out46) -> bram18/2
  debus_we/19(out46) -> bram18/3
  debus_addr/20(out45) -> bram19/1
  debus_din/20(out45) -> bram19/2
  debus_we/20(out45) -> bram19/3
  debus_addr/21(out44) -> bram20/1
  debus_din/21(out44) -> bram20/2
  debus_we/21(out44) -> bram20/3
  debus_addr/22(out43) -> bram21/1
  debus_din/22(out43) -> bram21/2
  debus_we/22(out43) -> bram21/3
  debus_addr/23(out42) -> bram22/1
  debus_din/23(out42) -> bram22/2
  debus_we/23(out42) -> bram22/3
  debus_addr/24(out41) -> bram23/1
  debus_din/24(out41) -> bram23/2
  debus_we/24(out41) -> bram23/3
  debus_addr/25(out40) -> bram24/1
  debus_din/25(out40) -> bram24/2
  debus_we/25(out40) -> bram24/3
  debus_addr/26(out39) -> bram25/1
  debus_din/26(out39) -> bram25/2
  debus_we/26(out39) -> bram25/3
  debus_addr/27(out38) -> bram26/1
  debus_din/27(out38) -> bram26/2
  debus_we/27(out38) -> bram26/3
  debus_addr/28(out37) -> bram27/1
  debus_din/28(out37) -> bram27/2
  debus_we/28(out37) -> bram27/3
  debus_addr/29(out36) -> bram28/1
  debus_din/29(out36) -> bram28/2
  debus_we/29(out36) -> bram28/3
  debus_addr/30(out35) -> bram29/1
  debus_din/30(out35) -> bram29/2
  debus_we/30(out35) -> bram29/3
  debus_addr/31(out34) -> bram30/1
  debus_din/31(out34) -> bram30/2
  debus_we/31(out34) -> bram30/3
  debus_addr/32(out33) -> bram31/1
  debus_din/32(out33) -> bram31/2
  debus_we/32(out33) -> bram31/3
  debus_addr/33(out32) -> bram32/1
  debus_din/33(out32) -> bram32/2
  debus_we/33(out32) -> bram32/3
  debus_addr/34(out31) -> bram33/1
  debus_din/34(out31) -> bram33/2
  debus_we/34(out31) -> bram33/3
  debus_addr/35(out30) -> bram34/1
  debus_din/35(out30) -> bram34/2
  debus_we/35(out30) -> bram34/3
  debus_addr/36(out29) -> bram35/1
  debus_din/36(out29) -> bram35/2
  debus_we/36(out29) -> bram35/3
  debus_addr/37(out28) -> bram36/1
  debus_din/37(out28) -> bram36/2
  debus_we/37(out28) -> bram36/3
  debus_addr/38(out27) -> bram37/1
  debus_din/38(out27) -> bram37/2
  debus_we/38(out27) -> bram37/3
  debus_addr/39(out26) -> bram38/1
  debus_din/39(out26) -> bram38/2
  debus_we/39(out26) -> bram38/3
  debus_addr/40(out25) -> bram39/1
  debus_din/40(out25) -> bram39/2
  debus_we/40(out25) -> bram39/3
  debus_addr/41(out24) -> bram40/1
  debus_din/41(out24) -> bram40/2
  debus_we/41(out24) -> bram40/3
  debus_addr/42(out23) -> bram41/1
  debus_din/42(out23) -> bram41/2
  debus_we/42(out23) -> bram41/3
  debus_addr/43(out22) -> bram42/1
  debus_din/43(out22) -> bram42/2
  debus_we/43(out22) -> bram42/3
  debus_addr/44(out21) -> bram43/1
  debus_din/44(out21) -> bram43/2
  debus_we/44(out21) -> bram43/3
  debus_addr/45(out20) -> bram44/1
  debus_din/45(out20) -> bram44/2
  debus_we/45(out20) -> bram44/3
  debus_addr/46(out19) -> bram45/1
  debus_din/46(out19) -> bram45/2
  debus_we/46(out19) -> bram45/3
  debus_addr/47(out18) -> bram46/1
  debus_din/47(out18) -> bram46/2
  debus_we/47(out18) -> bram46/3
  debus_addr/48(out17) -> bram47/1
  debus_din/48(out17) -> bram47/2
  debus_we/48(out17) -> bram47/3
  debus_addr/49(out16) -> bram48/1
  debus_din/49(out16) -> bram48/2
  debus_we/49(out16) -> bram48/3
  debus_addr/50(out15) -> bram49/1
  debus_din/50(out15) -> bram49/2
  debus_we/50(out15) -> bram49/3
  debus_addr/51(out14) -> bram50/1
  debus_din/51(out14) -> bram50/2
  debus_we/51(out14) -> bram50/3
  debus_addr/52(out13) -> bram51/1
  debus_din/52(out13) -> bram51/2
  debus_we/52(out13) -> bram51/3
  debus_addr/53(out12) -> bram52/1
  debus_din/53(out12) -> bram52/2
  debus_we/53(out12) -> bram52/3
  debus_addr/54(out11) -> bram53/1
  debus_din/54(out11) -> bram53/2
  debus_we/54(out11) -> bram53/3
  debus_addr/55(out10) -> bram54/1
  debus_din/55(out10) -> bram54/2
  debus_we/55(out10) -> bram54/3
  debus_addr/56(out9) -> bram55/1
  debus_din/56(out9) -> bram55/2
  debus_we/56(out9) -> bram55/3
  debus_addr/57(out8) -> bram56/1
  debus_din/57(out8) -> bram56/2
  debus_we/57(out8) -> bram56/3
  debus_addr/58(out7) -> bram57/1
  debus_din/58(out7) -> bram57/2
  debus_we/58(out7) -> bram57/3
  debus_addr/59(out6) -> bram58/1
  debus_din/59(out6) -> bram58/2
  debus_we/59(out6) -> bram58/3
  debus_addr/60(out5) -> bram59/1
  debus_din/60(out5) -> bram59/2
  debus_we/60(out5) -> bram59/3
  debus_addr/61(out4) -> bram60/1
  debus_din/61(out4) -> bram60/2
  debus_we/61(out4) -> bram60/3
  debus_addr/62(out3) -> bram61/1
  debus_din/62(out3) -> bram61/2
  debus_we/62(out3) -> bram61/3
  debus_addr/63(out2) -> bram62/1
  debus_din/63(out2) -> bram62/2
  debus_we/63(out2) -> bram62/3
  debus_addr/64(lsb_out1) -> bram63/1
  debus_din/64(lsb_out1) -> bram63/2
  debus_we/64(lsb_out1) -> bram63/3
  bram0/1 -> din_bussify/1(in1)
  bram1/1 -> din_bussify/2(in2)
  bram2/1 -> din_bussify/3(in3)
  bram3/1 -> din_bussify/4(in4)
  bram4/1 -> din_bussify/5(in5)
  bram5/1 -> din_bussify/6(in6)
  bram6/1 -> din_bussify/7(in7)
  bram7/1 -> din_bussify/8(in8)
  bram8/1 -> din_bussify/9(in9)
  bram9/1 -> din_bussify/10(in10)
  bram10/1 -> din_bussify/11(in11)
  bram11/1 -> din_bussify/12(in12)
  bram12/1 -> din_bussify/13(in13)
  bram13/1 -> din_bussify/14(in14)
  bram14/1 -> din_bussify/15(in15)
  bram15/1 -> din_bussify/16(in16)
  bram16/1 -> din_bussify/17(in17)
  bram17/1 -> din_bussify/18(in18)
  bram18/1 -> din_bussify/19(in19)
  bram19/1 -> din_bussify/20(in20)
  bram20/1 -> din_bussify/21(in21)
  bram21/1 -> din_bussify/22(in22)
  bram22/1 -> din_bussify/23(in23)
  bram23/1 -> din_bussify/24(in24)
  bram24/1 -> din_bussify/25(in25)
  bram25/1 -> din_bussify/26(in26)
  bram26/1 -> din_bussify/27(in27)
  bram27/1 -> din_bussify/28(in28)
  bram28/1 -> din_bussify/29(in29)
  bram29/1 -> din_bussify/30(in30)
  bram30/1 -> din_bussify/31(in31)
  bram31/1 -> din_bussify/32(in32)
  bram32/1 -> din_bussify/33(in33)
  bram33/1 -> din_bussify/34(in34)
  bram34/1 -> din_bussify/35(in35)
  bram35/1 -> din_bussify/36(in36)
  bram36/1 -> din_bussify/37(in37)
  bram37/1 -> din_bussify/38(in38)
  bram38/1 -> din_bussify/39(in39)
  bram39/1 -> din_bussify/40(in40)
  bram40/1 -> din_bussify/41(in41)
  bram41/1 -> din_bussify/42(in42)
  bram42/1 -> din_bussify/43(in43)
  bram43/1 -> din_bussify/44(in44)
  bram44/1 -> din_bussify/45(in45)
  bram45/1 -> din_bussify/46(in46)
  bram46/1 -> din_bussify/47(in47)
  bram47/1 -> din_bussify/48(in48)
  bram48/1 -> din_bussify/49(in49)
  bram49/1 -> din_bussify/50(in50)
  bram50/1 -> din_bussify/51(in51)
  bram51/1 -> din_bussify/52(in52)
  bram52/1 -> din_bussify/53(in53)
  bram53/1 -> din_bussify/54(in54)
  bram54/1 -> din_bussify/55(in55)
  bram55/1 -> din_bussify/56(in56)
  bram56/1 -> din_bussify/57(in57)
  bram57/1 -> din_bussify/58(in58)
  bram58/1 -> din_bussify/59(in59)
  bram59/1 -> din_bussify/60(in60)
  bram60/1 -> din_bussify/61(in61)
  bram61/1 -> din_bussify/62(in62)
  bram62/1 -> din_bussify/63(in63)
  bram63/1 -> din_bussify/64(in64)
  din_bussify/1(bus_out) -> dout/1
